simulink model "TwoPIDsimulink"  (R2021a)
settings: Solver=VariableStepAuto  StartTime=0.0  StopTime=100  RelTol=1e-3
values from neighbouring files (symbols this model uses):
  Ad = sysd.A    [FirstPoints.m]    (also in FirstProject.m; LQG.m; LQG3x3.m; LQR2x2.m)
  Bd = sysd.B    [FirstPoints.m]    (also in FirstProject.m; LQG.m; LQG3x3.m; LQR2x2.m)
  C = eye(2)    [FirstPoints.m]    (also in FirstProject.m; LQG.m = [1 0]; LQG3x3.m = eye(3); LQR3x3.m = eye(3))
  D = zeros(2, 1)    [FirstPoints.m]    (also in FirstProject.m; LQG.m; LQG3x3.m = zeros(3, 2); LQR3x3.m = zeros(3,2))
  sampleTime = 0.1    [FirstPoints.m]    (also in FirstProject.m; LQG.m = 1; LQG3x3.m = 1; LQR2x2.m = 1)
  x0 = [1 ... (first row only)    [FirstPoints.m]    (also in FirstProject.m; LQG.m = [1 1]'; LQG3x3.m = [10 -2 5]'; LQR2x2.m = [10)
libraries: pid_lib x1
settings Model: Creator=lukar  LastModifiedBy=lukar

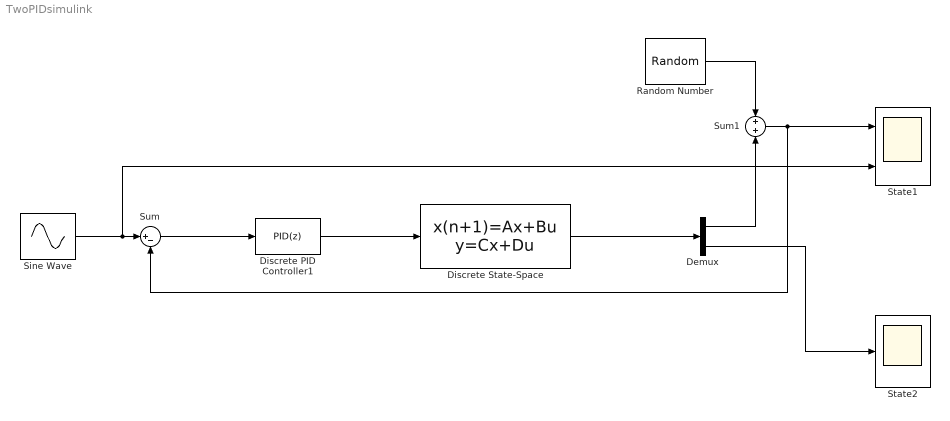
== system TwoPIDsimulink ==
  Demux : Demux  Outputs=2
  Discrete PID Controller1 : pid_lib/PID Controller  Controller=PID  Form=Parallel  TimeDomain=Discrete-time  UseExternalTs=off  SampleTime=-1  IntegratorMethod=Forward Euler  FilterMethod=Forward Euler  ControllerParametersSource=internal  P=390  I=15  D=559  UseFilter=on  N=12.6590148265937  TunerSelectOption=Transfer Function Based (PID Tuner App)  InitialConditionSource=internal  InitialConditionForIntegrator=0  InitialConditionForFilter=0  DifferentiatorICPrevScaledInput=0  ExternalReset=none  TrackingMode=off  Kt=1  LimitOutput=off  SatLimitsSource=internal  UpperSaturationLimit=inf  LowerSaturationLimit=-inf  LinearizeAsGain=off  AntiWindupMode=none  Kb=1  POutMin=[]  POutMax=[]  IOutMin=[]  IOutMax=[]  DOutMin=[]  DOutMax=[]  NOutMin=[]  NOutMax=[]  SumOutMin=[]  SumOutMax=[]  SaturationOutMin=[]  SaturationOutMax=[]  PParamMin=[]  PParamMax=[]  IParamMin=[]  IParamMax=[]  DParamMin=[]  DParamMax=[]  NParamMin=[]  NParamMax=[]  KbParamMin=[]  KbParamMax=[]  KtParamMin=[]  KtParamMax=[]  KbOutMin=[]  KbOutMax=[]  KtOutMin=[]  KtOutMax=[]  IntegratorOutMin=[]  IntegratorOutMax=[]  FilterOutMin=[]  FilterOutMax=[]  SumI1OutMin=[]  SumI1OutMax=[]  SumI2OutMin=[]  SumI2OutMax=[]  SumI3OutMin=[]  SumI3OutMax=[]  SumI4OutMin=[]  SumI4OutMax=[]  SumDOutMin=[]  SumDOutMax=[]  DifferentiatorOutMin=[]  DifferentiatorOutMax=[]  FilterDiffOutCoefMin=[]  FilterDiffOutCoefMax=[]  ReciprocalOutMin=[]  ReciprocalOutMax=[]  SumDenOutMin=[]  SumDenOutMax=[]  SumNumOutMin=[]  SumNumOutMax=[]  DivideOutMin=[]  DivideOutMax=[]  UdiffTsProdOutMin=[]  UdiffTsProdOutMax=[]  NTsProdOutMin=[]  NTsProdOutMax=[]  UintegralTsProdOutMin=[]  UintegralTsProdOutMax=[]  UngainTsProdOutMin=[]  UngainTsProdOutMax=[]  IntegratorContinuousStateAttributes=''  IntegratorStateMustResolveToSignalObject=off  IntegratorRTWStateStorageClass=Auto  FilterContinuousStateAttributes=''  FilterStateMustResolveToSignalObject=off  FilterRTWStateStorageClass=Auto  ParallelPVariant=InternalParameters  IdealPVariant=Disabled  IVariant=InternalParameters  DVariant=InternalParameters  IntegratorVariant=Discrete  SatVariant=Disabled  AWVariant=Passthrough  PCopyVariant=Disabled  TRVariant=Disabled  FdbkBlocksVariant=Forward  IdealPFdbkVariant=Disabled  SatFdbkVariant=Disabled  DerivativeFilterVariant=ForwardEulerFilter  NVariant=InternalParameters  NCopyVariant=Disabled  FilterICVariant=InternalICsFilter  IntegratorICVariant=InternalICs  ExternalResetVariant=Disabled  TRSumVariant=Passthrough  SumFdbkVariant=Disabled  SumVariant=Sum_PID  TsampFilterVariant=InternalTs  TsampNgainVariant=Passthrough  TsampIntegralVariant=Passthrough  ExternalSaturationOutDataTypeStr=Inherit: Same as second input
  Discrete State-Space : DiscreteStateSpace  A=Ad  B=Bd  C=C  D=D  InitialCondition=x0  SampleTime=sampleTime
  Random Number : RandomNumber  Variance=0.1  SampleTime=sampleTime
  Sine Wave : Sin  Amplitude=4  SampleTime=sampleTime
  State1 : Scope  NumInputPorts=2
  State2 : Scope
  Sum : Sum  Inputs=|+-
  Sum1 : Sum  Inputs=+|+
  wires:
  Discrete State-Space/1 -> Demux/1
  Sine Wave/1 -> State1/2, Sum/1
  Demux/2 -> State2/1
  Demux/1 -> Sum1/2
  Random Number/1 -> Sum1/1
  Sum1/1 -> Sum/2, State1/1
  Sum/1 -> Discrete PID Controller1/1
  Discrete PID Controller1/1 -> Discrete State-Space/1
